simulink model "Sample"  (R2018b)
settings: Solver=FixedStepAuto  StartTime=0.0  StopTime=10.0  FixedStep=0.1  RelTol=1e-3
settings Model: Creator=Amir  LastModifiedBy=Amir

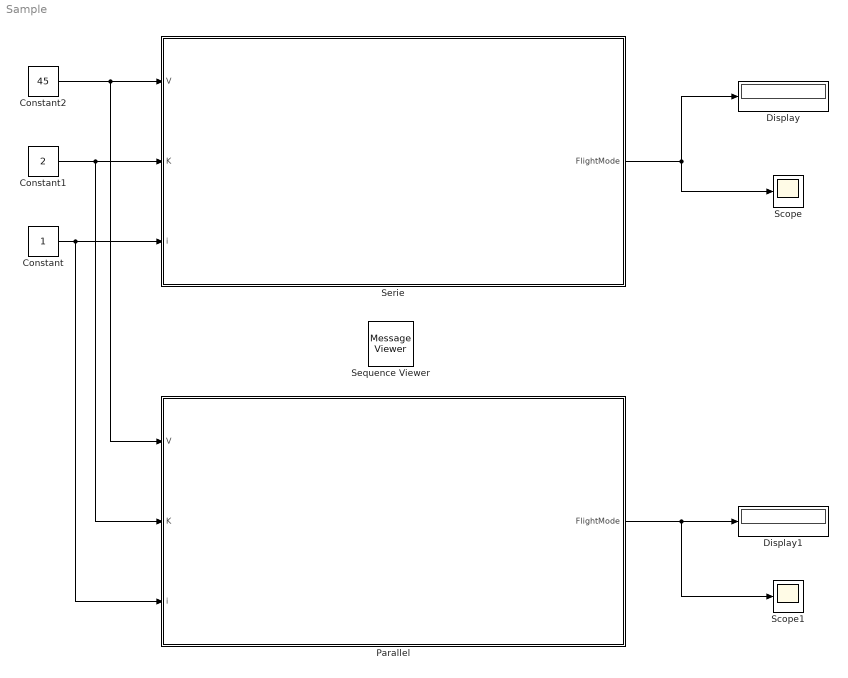
== system Sample ==
  Constant : Constant
  Constant1 : Constant  Value=2
  Constant2 : Constant  Value=45
  Display : Display
  Display1 : Display
  Parallel : Stateflow chart  TreatAsAtomicUnit=on
  Scope : Scope
  Scope1 : Scope
  Sequence Viewer : MessageViewer
  Serie : Stateflow chart  TreatAsAtomicUnit=on
  wires:
  Serie/1(FlightMode) -> Display/1, Scope/1
  Constant/1 -> Parallel/3(i), Serie/3(i)
  Constant1/1 -> Parallel/2(K), Serie/2(K)
  Constant2/1 -> Parallel/1(V), Serie/1(V)
  Parallel/1(FlightMode) -> Scope1/1, Display1/1

== stateflow chart Sample/Parallel ==
  state WaypointTrack [parallel]
    if i==1
    FlightMode=2;
    else
    FlightMode=5;
    end
    settings: executionOrder=1
  state Loiter [parallel]
    if i==2
    FlightMode=3;
    else
    FlightMode=8;
    end
    settings: executionOrder=2
  state Return2Base [parallel]
    if i==3
    FlightMode=4;
    else
    FlightMode=6;
    end
    settings: executionOrder=3
  data: FlightMode output; V input; K input; i input

== stateflow chart Sample/Serie ==
  state WaypointTrack
    if i==1
    FlightMode=2;
    else
    FlightMode=5;
    end
  state Loiter
    if i==1
    FlightMode=3;
    else
    FlightMode=8;
    end
  state Return2Base
    if i==1
    FlightMode=4;
    else
    FlightMode=6;
    end
  (default) -> WaypointTrack
  WaypointTrack -> Loiter [order 1] : [V>=40]
  Loiter -> WaypointTrack [order 1] : [V<40]
  Return2Base -> WaypointTrack [order 1] : [V>=50]
  WaypointTrack -> Return2Base [order 2] : [V<30]
  Loiter -> Return2Base [order 2] : [K==2]
  Return2Base -> Loiter [order 2] : [K~=2]
  data: FlightMode output; V input; K input; i input
